simulink model "mag_pd_control_test"  (R2016b)
settings: Solver=VariableStepAuto  StartTime=0.0  StopTime=360  RelTol=1e-3
values from neighbouring files (symbols this model uses):
  omega_cmd = zeros(3,1)    [mag_pd_control_IC_test.m]    (also in mag_pd_control_gain_test_init.m; mag_pd_control_test_init.m)
  quat_cmd = [1;0;0;0]    [mag_pd_control_IC_test.m]    (also in mag_pd_control_gain_test_init.m; mag_pd_control_test_init.m)
undefined symbols (not defined in the file or in its folder): fsw_params
libraries: dynamics_lib x2, vrlib x1, GPS_time_lib x1, mag_PD_control_new x1, mag_vec_LS_lib x1, mag_vec_lib x1, magnetometer_lib x1, magnetorquer_assembly_lib x1, sgp4_lib_fsw x1, time_coord_rotation_lib x1
settings Model: Creator=taylorreynolds  LastModifiedBy=bijan

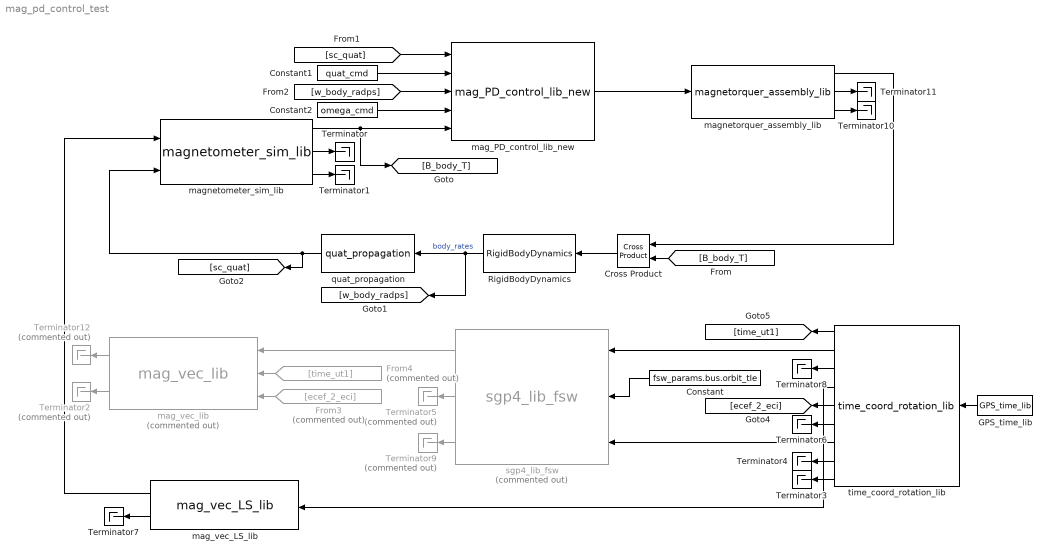
== system mag_pd_control_test ==
  Constant : Constant  Value=fsw_params.bus.orbit_tle
  Constant1 : Constant  Value=quat_cmd
  Constant2 : Constant  Value=omega_cmd
  Cross Product : vrlib/Utilities/Cross Product
  From3 : From  Commented=on  GotoTag=ecef_2_eci
  From4 : From  Commented=on  GotoTag=time_ut1
  GPS_time_lib : GPS_time_lib/GPS_time_lib
  RigidBodyDynamics : dynamics_lib/Dynamics/RigidBodyDynamics
  Terminator{,1,3..4,6..8,10..11} (9 alike) : Terminator
  Terminator{2,5,9,12} (4 alike) : Terminator  Commented=on
  "mag_PD_control_lib_new " : mag_PD_control_new/mag_PD_control_lib_new 
  mag_vec_LS_lib : mag_vec_LS_lib/mag_vec_LS_lib
  mag_vec_lib : mag_vec_lib/mag_vec_lib  Commented=on
  magnetometer_sim_lib : magnetometer_lib/magnetometer_sim_lib  seed_x=4  seed_y=5  seed_z=6
  magnetorquer_assembly_lib : magnetorquer_assembly_lib/magnetorquer_assembly_lib
  quat_propagation : dynamics_lib/Dynamics/quat_propagation
  sgp4_lib_fsw : sgp4_lib_fsw/sgp4_lib_fsw  Commented=on
  time_coord_rotation_lib : time_coord_rotation_lib/time_coord_rotation_lib
  wires:
  RigidBodyDynamics/1 -> [w_body_radps], quat_propagation/1  "body_rates"
  "mag_PD_control_lib_new "/1 -> magnetorquer_assembly_lib/1
  magnetometer_sim_lib/1 -> "mag_PD_control_lib_new "/5, [B_body_T]
  quat_propagation/1 -> [sc_quat], magnetometer_sim_lib/2
  magnetometer_sim_lib/2 -> Terminator/1
  magnetometer_sim_lib/3 -> Terminator1/1
  mag_vec_lib/2 -> Terminator2/1
  GPS_time_lib/1 -> time_coord_rotation_lib/1
  time_coord_rotation_lib/9 -> Terminator3/1
  time_coord_rotation_lib/8 -> Terminator4/1
  time_coord_rotation_lib/6 -> Terminator6/1
  time_coord_rotation_lib/3 -> Terminator8/1
  magnetorquer_assembly_lib/3 -> Terminator10/1
  magnetorquer_assembly_lib/2 -> Terminator11/1
  Constant/1 -> sgp4_lib_fsw/2
  magnetorquer_assembly_lib/1 -> Cross Product/1
  Cross Product/1 -> RigidBodyDynamics/1
  Constant2/1 -> "mag_PD_control_lib_new "/4
  [sc_quat] -> "mag_PD_control_lib_new "/1
  [w_body_radps] -> "mag_PD_control_lib_new "/3
  time_coord_rotation_lib/7 -> sgp4_lib_fsw/3
  time_coord_rotation_lib/5 -> [ecef_2_eci]
  time_coord_rotation_lib/1 -> [time_ut1]
  time_coord_rotation_lib/2 -> sgp4_lib_fsw/1
  From3/1 -> mag_vec_lib/3
  From4/1 -> mag_vec_lib/2
  sgp4_lib_fsw/1 -> mag_vec_lib/1
  sgp4_lib_fsw/2 -> Terminator5/1
  sgp4_lib_fsw/3 -> Terminator9/1
  Constant1/1 -> "mag_PD_control_lib_new "/2
  time_coord_rotation_lib/4 -> mag_vec_LS_lib/1
  mag_vec_LS_lib/2 -> Terminator7/1
  mag_vec_LS_lib/1 -> magnetometer_sim_lib/1
  mag_vec_lib/1 -> Terminator12/1
  [B_body_T] -> Cross Product/2
